simulink model "SrmMatlabZzh1"  (Simulink 7.3)
settings: Solver=ode45  StartTime=0.0  StopTime=10.0  RelTol=1e-3
libraries: powerlib x27, powerlib_extras x1
settings Model: Creator=Administrator  LastModifiedBy=Think79

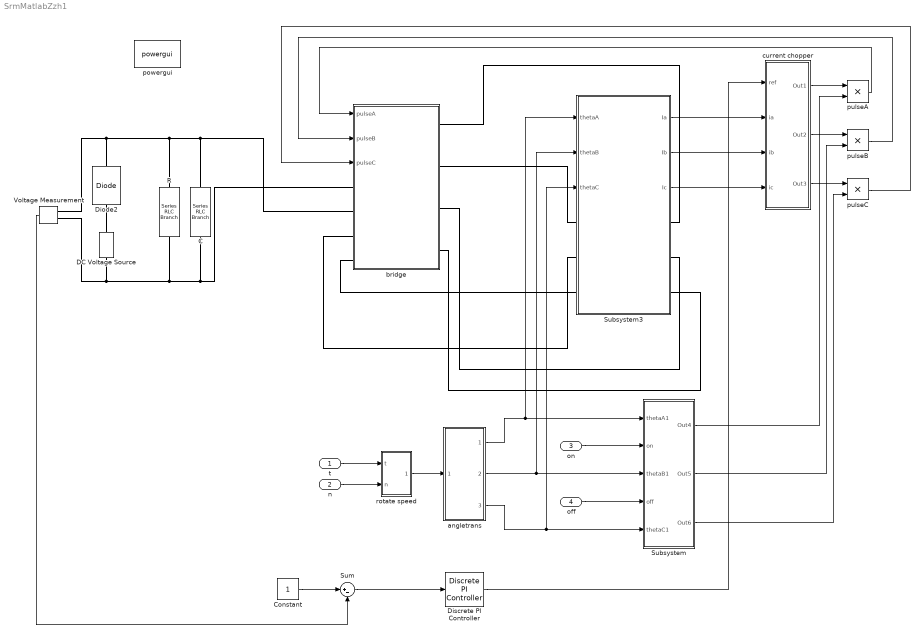
== system SrmMatlabZzh1 ==
  t : Inport  OutDataType=fixdt(1, 16)  OutScaling=2^0
  n : Inport  Port=2  OutDataType=fixdt(1, 16)  OutScaling=2^0
  on : Inport  Port=3  OutDataType=fixdt(1, 16)  OutScaling=2^0
  off : Inport  Port=4  OutDataType=fixdt(1, 16)  OutScaling=2^0
  "C " : powerlib/Elements/Series RLC Branch  DialogController=POWERSYS.PowerSysDialog  PhysicalDomain=powersysdomain  SubClassName=unknown  LeftPortType=p1  RightPortType=p1  LConnTagsString=__new0  RConnTagsString=__new0  BranchType=C  Resistance=1  Inductance=1.0  SetiL0=off  InitialCurrent=0  Capacitance=1e-3  Setx0=off  InitialVoltage=0  Measurements=None
  Constant : Constant  OutDataType=fixdt(1, 16)  OutScaling=2^0
  DC Voltage Source : powerlib/Electrical Sources/DC Voltage Source  DialogController=POWERSYS.PowerSysDialog  SystemSampleTime=-1  Amplitude=60  Measurements=None
  Diode2 : powerlib/Power Electronics/Diode  DialogController=POWERSYS.PowerSysDialog  SystemSampleTime=-1  Ron=0.001  Lon=0  Vf=0.8  IC=0  UseSnubber=off  Rs=500  Cs=250e-9  Measurements=off
  Discrete PI Controller : powerlib_extras/Discrete  Control Blocks/Discrete PI Controller  DialogController=POWERSYS.PowerSysDialog  SystemSampleTime=-1  Kp=0.1  Ki=1  Par_Limits=[1e6 -1e6]  Init=0  Ts=50e-6
  R : powerlib/Elements/Series RLC Branch  DialogController=POWERSYS.PowerSysDialog  PhysicalDomain=powersysdomain  SubClassName=unknown  LeftPortType=p1  RightPortType=p1  LConnTagsString=__new0  RConnTagsString=__new0  BranchType=R  Resistance=1  Inductance=1.0  SetiL0=off  InitialCurrent=0  Capacitance=1.0  Setx0=off  InitialVoltage=0  Measurements=None
  Subsystem : Subsystem
  Subsystem3 : Subsystem
  Sum : Sum  Inputs=|+-  OutDataType=fixdt(1, 16)  OutScaling=2^0
  Voltage Measurement : powerlib/Measurements/Voltage Measurement  DialogController=POWERSYS.PowerSysDialog  SystemSampleTime=-1  PhasorSimulation=off  OutputType=Complex  PSBequivalent=0
  angletrans : Subsystem
  bridge : Subsystem
  current chopper : Subsystem
  powergui : powerlib/powergui  Priority=1  SystemSampleTime=-1  SimulationMode=Continuous  SampleTime=50e-6  frequency=60  SPID=off  DisableSnubberDevices=off  DisableRonSwitches=off  DisableVfSwitches=off  SwTol=0  Interpol=off  frequencyindice=0  echomessages=off  HookPort=off  DisplayEquations=off  FunctionMessages=off  EnableUseOfTLC=off  x0status=blocks  RestoreLinks=warning  Frange=[0:2:500]  Ylog=off  Xlog=on  ShowGrid=off  save=off  variable=ZData  ZoomFFT=on  StartTime=0.0  cycles=1  DisplayStyle=1  fundamental=60  FreqAxis=off  MaxFrequency=1000  frequencyindicesteady=1  RmsSteady=1  display=off  Ts=0  methode=off
  pulseA : Product  OutDataType=fixdt(1, 16)  OutScaling=2^0  RndMeth=Zero
  pulseB : Product  OutDataType=fixdt(1, 16)  OutScaling=2^0  RndMeth=Zero
  pulseC : Product  OutDataType=fixdt(1, 16)  OutScaling=2^0  RndMeth=Zero
  rotate speed : Subsystem
  wires:
  Subsystem3/1(Ia) -> current chopper/2(ia)
  Subsystem3/2(Ib) -> current chopper/3(ib)
  Subsystem3/3(Ic) -> current chopper/4(ic)
  rotate speed/1(theta) -> angletrans/1(theta)
  t/1 -> rotate speed/1(t)
  n/1 -> rotate speed/2(n)
  on/1 -> Subsystem/2(on)
  off/1 -> Subsystem/4(off)
  angletrans/1(thetaA) -> Subsystem/1(thetaA1), Subsystem3/1(thetaA)
  angletrans/2(thetaB) -> Subsystem/3(thetaB1), Subsystem3/2(thetaB)
  angletrans/3(thetaC) -> Subsystem/5(thetaC1), Subsystem3/3(thetaC)
  Voltage Measurement/1 -> Sum/2
  Sum/1 -> Discrete PI Controller/1
  Constant/1 -> Sum/1
  Discrete PI Controller/1 -> current chopper/1(ref)
  Subsystem/1(Out4) -> pulseA/2
  Subsystem/3(Out6) -> pulseC/2
  Subsystem/2(Out5) -> pulseB/2
  current chopper/1(Out1) -> pulseA/1
  current chopper/2(Out2) -> pulseB/1
  current chopper/3(Out3) -> pulseC/1
  pulseB/1 -> bridge/2(pulseB)
  pulseC/1 -> bridge/3(pulseC)
  pulseA/1 -> bridge/1(pulseA)
  connections:
  Diode2/LConn1 -- DC Voltage Source/RConn1
  Diode2/RConn1 -- R/LConn1 -- "C "/RConn1 -- bridge/LConn2 -- Voltage Measurement/LConn1
  "C "/LConn1 -- bridge/LConn1 -- R/RConn1 -- DC Voltage Source/LConn1 -- Voltage Measurement/LConn2
  bridge/RConn2 -- Subsystem3/LConn1
  bridge/RConn1 -- Subsystem3/RConn1
  bridge/LConn3 -- Subsystem3/LConn2
  bridge/LConn4 -- Subsystem3/LConn3
  bridge/RConn4 -- Subsystem3/RConn3
  bridge/RConn3 -- Subsystem3/RConn2

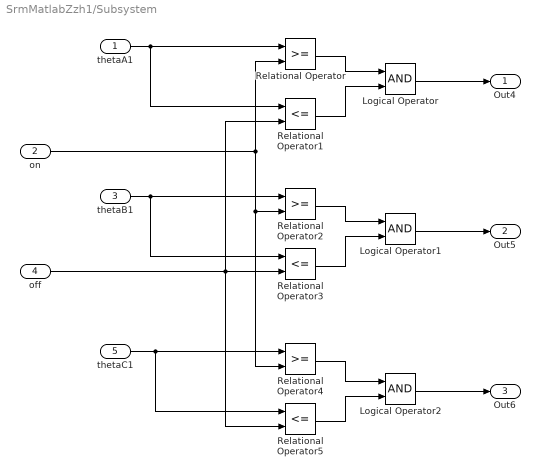
== system SrmMatlabZzh1/Subsystem ==
  thetaA1 : Inport  OutDataType=fixdt(1, 16)  OutScaling=2^0
  on : Inport  Port=2  OutDataType=fixdt(1, 16)  OutScaling=2^0
  thetaB1 : Inport  Port=3  OutDataType=fixdt(1, 16)  OutScaling=2^0
  off : Inport  Port=4  OutDataType=fixdt(1, 16)  OutScaling=2^0
  thetaC1 : Inport  Port=5  OutDataType=fixdt(1, 16)  OutScaling=2^0
  Logical Operator : Logic  AllPortsSameDT=off  OutDataTypeMode=boolean  LogicDataType=fixdt(0, 8)  OutDataTypeStr=boolean
  Logical Operator1 : Logic  AllPortsSameDT=off  OutDataTypeMode=boolean  LogicDataType=fixdt(0, 8)  OutDataTypeStr=boolean
  Logical Operator2 : Logic  AllPortsSameDT=off  OutDataTypeMode=boolean  LogicDataType=fixdt(0, 8)  OutDataTypeStr=boolean
  Relational Operator : RelationalOperator  LogicOutDataTypeMode=boolean  LogicDataType=fixdt(0, 8)  OutDataTypeStr=boolean
  Relational Operator1 : RelationalOperator  Operator=<=  LogicOutDataTypeMode=boolean  LogicDataType=fixdt(0, 8)  OutDataTypeStr=boolean
  Relational Operator2 : RelationalOperator  LogicOutDataTypeMode=boolean  LogicDataType=fixdt(0, 8)  OutDataTypeStr=boolean
  Relational Operator3 : RelationalOperator  Operator=<=  LogicOutDataTypeMode=boolean  LogicDataType=fixdt(0, 8)  OutDataTypeStr=boolean
  Relational Operator4 : RelationalOperator  LogicOutDataTypeMode=boolean  LogicDataType=fixdt(0, 8)  OutDataTypeStr=boolean
  Relational Operator5 : RelationalOperator  Operator=<=  LogicOutDataTypeMode=boolean  LogicDataType=fixdt(0, 8)  OutDataTypeStr=boolean
  Out4 : Outport  OutDataType=fixdt(1, 16)  OutScaling=2^0
  Out5 : Outport  Port=2  OutDataType=fixdt(1, 16)  OutScaling=2^0
  Out6 : Outport  Port=3  OutDataType=fixdt(1, 16)  OutScaling=2^0
  wires:
  thetaA1/1 -> Relational Operator/1, Relational Operator1/1
  thetaB1/1 -> Relational Operator2/1, Relational Operator3/1
  thetaC1/1 -> Relational Operator4/1, Relational Operator5/1
  on/1 -> Relational Operator/2, Relational Operator2/2, Relational Operator4/2
  off/1 -> Relational Operator1/2, Relational Operator3/2, Relational Operator5/2
  Relational Operator/1 -> Logical Operator/1
  Relational Operator1/1 -> Logical Operator/2
  Relational Operator2/1 -> Logical Operator1/1
  Relational Operator3/1 -> Logical Operator1/2
  Relational Operator4/1 -> Logical Operator2/1
  Relational Operator5/1 -> Logical Operator2/2
  Logical Operator/1 -> Out4/1
  Logical Operator1/1 -> Out5/1
  Logical Operator2/1 -> Out6/1

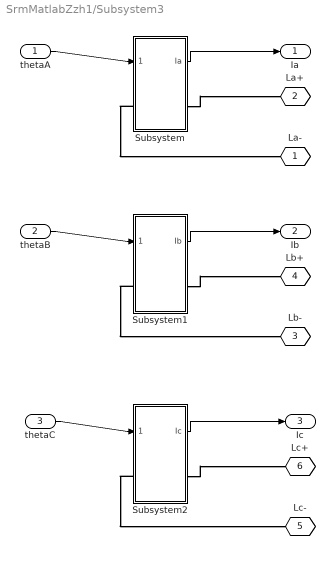
== system SrmMatlabZzh1/Subsystem3 ==
  thetaA : Inport  OutDataType=fixdt(1, 16)  OutScaling=2^0
  thetaB : Inport  Port=2  OutDataType=fixdt(1, 16)  OutScaling=2^0
  thetaC : Inport  Port=3  OutDataType=fixdt(1, 16)  OutScaling=2^0
  Subsystem : Subsystem
  Subsystem1 : Subsystem
  Subsystem2 : Subsystem
  La- : PMIOPort  Tag=PMCPort  Port=1  Side=Left
  La+ : PMIOPort  Tag=PMCPort  Port=2  Side=Right
  Lb- : PMIOPort  Tag=PMCPort  Port=3  Side=Left
  Lb+ : PMIOPort  Tag=PMCPort  Port=4  Side=Right
  Lc- : PMIOPort  Tag=PMCPort  Port=5  Side=Left
  Lc+ : PMIOPort  Tag=PMCPort  Port=6  Side=Right
  Ia : Outport  OutDataType=fixdt(1, 16)  OutScaling=2^0
  Ib : Outport  Port=2  OutDataType=fixdt(1, 16)  OutScaling=2^0
  Ic : Outport  Port=3  OutDataType=fixdt(1, 16)  OutScaling=2^0
  wires:
  thetaA/1 -> Subsystem/1(thetaA)
  Subsystem/1(Ia) -> Ia/1
  thetaB/1 -> Subsystem1/1(thetaB)
  Subsystem1/1(Ib) -> Ib/1
  thetaC/1 -> Subsystem2/1(thetaC)
  Subsystem2/1(Ic) -> Ic/1
  connections:
  Subsystem/LConn1 -- La-/RConn1
  Subsystem/RConn1 -- La+/RConn1
  Subsystem1/LConn1 -- Lb-/RConn1
  Subsystem1/RConn1 -- Lb+/RConn1
  Subsystem2/LConn1 -- Lc-/RConn1
  Subsystem2/RConn1 -- Lc+/RConn1

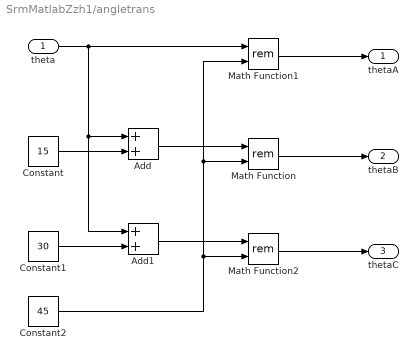
== system SrmMatlabZzh1/angletrans ==
  theta : Inport  OutDataType=fixdt(1, 16)  OutScaling=2^0
  Add : Sum  OutDataType=fixdt(1, 16)  OutScaling=2^-10
  Add1 : Sum  OutDataType=fixdt(1, 16)  OutScaling=2^-10
  Constant : Constant  Value=15  OutDataType=fixdt(1, 16)  OutScaling=2^0
  Constant1 : Constant  Value=30  OutDataType=fixdt(1, 16)  OutScaling=2^0
  Constant2 : Constant  Value=45  OutDataType=fixdt(1, 16)  OutScaling=2^0
  Math Function : Math  Operator=rem  OutDataType=fixdt(1, 16)  OutScaling=2^0  SaturateOnIntegerOverflow=on
  Math Function1 : Math  Operator=rem  OutDataType=fixdt(1, 16)  OutScaling=2^0  SaturateOnIntegerOverflow=on
  Math Function2 : Math  Operator=rem  OutDataType=fixdt(1, 16)  OutScaling=2^0  SaturateOnIntegerOverflow=on
  thetaA : Outport  OutDataType=fixdt(1, 16)  OutScaling=2^0
  thetaB : Outport  Port=2  OutDataType=fixdt(1, 16)  OutScaling=2^0
  thetaC : Outport  Port=3  OutDataType=fixdt(1, 16)  OutScaling=2^0
  wires:
  Add1/1 -> Math Function2/1
  Add/1 -> Math Function/1
  theta/1 -> Math Function1/1, Add1/1, Add/1
  Constant/1 -> Add/2
  Constant1/1 -> Add1/2
  Constant2/1 -> Math Function2/2, Math Function/2, Math Function1/2
  Math Function2/1 -> thetaC/1
  Math Function/1 -> thetaB/1
  Math Function1/1 -> thetaA/1

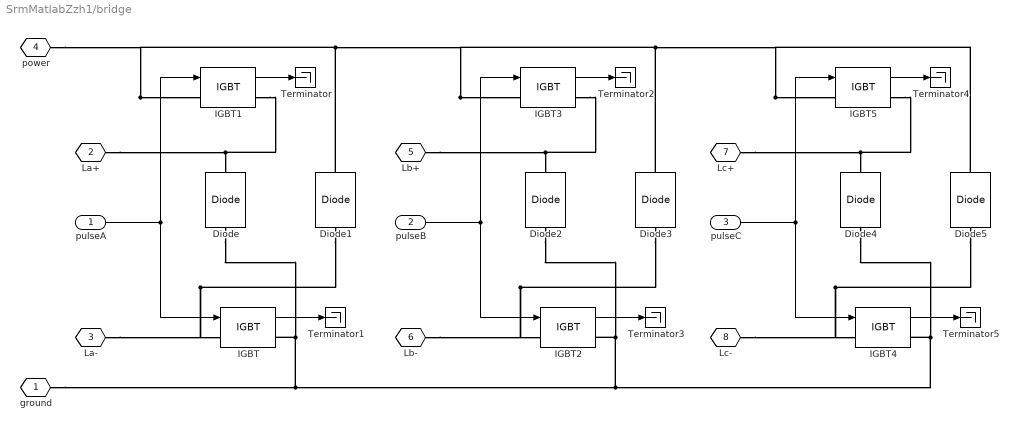
== system SrmMatlabZzh1/bridge ==
  pulseA : Inport  OutDataType=fixdt(1, 16)  OutScaling=2^0
  pulseB : Inport  Port=2  OutDataType=fixdt(1, 16)  OutScaling=2^0
  pulseC : Inport  Port=3  OutDataType=fixdt(1, 16)  OutScaling=2^0
  Diode{,1..5} (6 alike) : powerlib/Power Electronics/Diode  DialogController=POWERSYS.PowerSysDialog  SystemSampleTime=-1  Ron=0.001  Lon=0  Vf=0.8  IC=0  UseSnubber=off  Rs=500  Cs=250e-9  Measurements=off
  IGBT{,1..5} (6 alike) : powerlib/Power Electronics/IGBT  DialogController=POWERSYS.PowerSysDialog  SystemSampleTime=-1  Ron=0.001  Lon=0  Vf=1  Tf=1e-6  Tt=2e-6  IC=0  Rs=1e5  Cs=inf  Measurements=on
  Terminator{,1..5} (6 alike) : Terminator
  ground : PMIOPort  Tag=PMCPort  Port=1  Side=Left
  La+ : PMIOPort  Tag=PMCPort  Port=2  Side=Right
  La- : PMIOPort  Tag=PMCPort  Port=3  Side=Right
  power : PMIOPort  Tag=PMCPort  Port=4  Side=Left
  Lb+ : PMIOPort  Tag=PMCPort  Port=5  Side=Right
  Lb- : PMIOPort  Tag=PMCPort  Port=6  Side=Left
  Lc+ : PMIOPort  Tag=PMCPort  Port=7  Side=Right
  Lc- : PMIOPort  Tag=PMCPort  Port=8  Side=Left
  wires:
  IGBT4/1 -> Terminator5/1
  IGBT5/1 -> Terminator4/1
  pulseC/1 -> IGBT4/1, IGBT5/1
  IGBT2/1 -> Terminator3/1
  IGBT3/1 -> Terminator2/1
  pulseB/1 -> IGBT2/1, IGBT3/1
  IGBT/1 -> Terminator1/1
  IGBT1/1 -> Terminator/1
  pulseA/1 -> IGBT/1, IGBT1/1
  connections:
  Lc-/RConn1 -- IGBT4/LConn1 -- Diode5/LConn1
  Lc+/RConn1 -- IGBT5/RConn1 -- Diode4/RConn1
  Lb-/RConn1 -- IGBT2/LConn1 -- Diode3/LConn1
  Lb+/RConn1 -- IGBT3/RConn1 -- Diode2/RConn1
  Diode5/RConn1 -- IGBT5/LConn1 -- Diode3/RConn1 -- IGBT3/LConn1 -- Diode1/RConn1 -- IGBT1/LConn1 -- power/RConn1
  La-/RConn1 -- IGBT/LConn1 -- Diode1/LConn1
  La+/RConn1 -- IGBT1/RConn1 -- Diode/RConn1
  IGBT2/RConn1 -- Diode2/LConn1 -- IGBT/RConn1 -- Diode/LConn1 -- ground/RConn1 -- IGBT4/RConn1 -- Diode4/LConn1

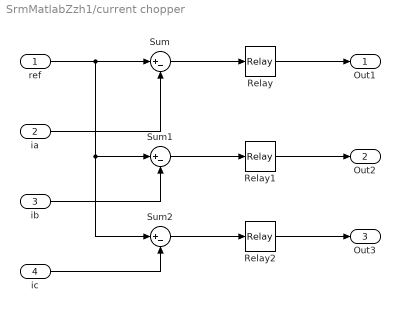
== system SrmMatlabZzh1/current chopper ==
  ref : Inport  OutDataType=fixdt(1, 16)  OutScaling=2^0
  ia : Inport  Port=2  OutDataType=fixdt(1, 16)  OutScaling=2^0
  ib : Inport  Port=3  OutDataType=fixdt(1, 16)  OutScaling=2^0
  ic : Inport  Port=4  OutDataType=fixdt(1, 16)  OutScaling=2^0
  Relay : Relay  OutDataType=fixdt(1, 16)  OutScaling=2^0
  Relay1 : Relay  OutDataType=fixdt(1, 16)  OutScaling=2^0
  Relay2 : Relay  OutDataType=fixdt(1, 16)  OutScaling=2^0
  Sum : Sum  Inputs=|+-  OutDataType=fixdt(1, 16)  OutScaling=2^0
  Sum1 : Sum  Inputs=|+-  OutDataType=fixdt(1, 16)  OutScaling=2^0
  Sum2 : Sum  Inputs=|+-  OutDataType=fixdt(1, 16)  OutScaling=2^0
  Out1 : Outport  OutDataType=fixdt(1, 16)  OutScaling=2^0
  Out2 : Outport  Port=2  OutDataType=fixdt(1, 16)  OutScaling=2^0
  Out3 : Outport  Port=3  OutDataType=fixdt(1, 16)  OutScaling=2^0
  wires:
  Relay/1 -> Out1/1
  Relay1/1 -> Out2/1
  Relay2/1 -> Out3/1
  Sum/1 -> Relay/1
  Sum1/1 -> Relay1/1
  Sum2/1 -> Relay2/1
  ref/1 -> Sum/1, Sum2/1, Sum1/1
  ia/1 -> Sum/2
  ib/1 -> Sum1/2
  ic/1 -> Sum2/2

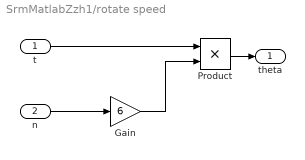
== system SrmMatlabZzh1/rotate speed ==
  t : Inport  OutDataType=fixdt(1, 16)  OutScaling=2^0
  n : Inport  Port=2  OutDataType=fixdt(1, 16)  OutScaling=2^0
  Gain : Gain  Gain=6  ParameterDataType=fixdt(1, 16)  ParameterScaling=2^0  OutDataType=fixdt(1, 16)  OutScaling=2^0
  Product : Product  OutDataType=fixdt(1, 16)  OutScaling=2^0  RndMeth=Zero
  theta : Outport
  wires:
  n/1 -> Gain/1
  Gain/1 -> Product/2
  t/1 -> Product/1
  Product/1 -> theta/1

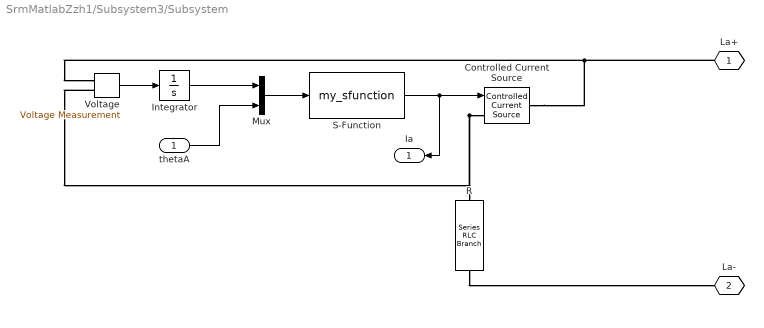
== system SrmMatlabZzh1/Subsystem3/Subsystem ==
  thetaA : Inport  OutDataType=fixdt(1, 16)  OutScaling=2^0
  Controlled Current Source : powerlib/Electrical Sources/Controlled Current Source  DialogController=POWERSYS.PowerSysDialog  SystemSampleTime=-1  Initialize=on  Source_Type=AC  Amplitude=0  Phase=0  Frequency=0  Measurements=None
  Integrator : Integrator
  Mux : Mux  Inputs=2
  R : powerlib/Elements/Series RLC Branch  DialogController=POWERSYS.PowerSysDialog  PhysicalDomain=powersysdomain  SubClassName=unknown  LeftPortType=p1  RightPortType=p1  LConnTagsString=__new0  RConnTagsString=__new0  BranchType=R  Resistance=0.0261014  Inductance=1.0  SetiL0=off  InitialCurrent=0  Capacitance=1.0  Setx0=off  InitialVoltage=0  Measurements=None
  S-Function : S-Function  FunctionName=my_sfunction  EnableBusSupport=off
  Voltage : powerlib/Measurements/Voltage Measurement  DialogController=POWERSYS.PowerSysDialog  SystemSampleTime=-1  PhasorSimulation=off  OutputType=Complex  PSBequivalent=0
  La+ : PMIOPort  Tag=PMCPort  Port=1  Side=Right
  La- : PMIOPort  Tag=PMCPort  Port=2  Side=Left
  Ia : Outport  OutDataType=fixdt(1, 16)  OutScaling=2^0
  wires:
  Mux/1 -> S-Function/1
  Integrator/1 -> Mux/1
  thetaA/1 -> Mux/2
  S-Function/1 -> Ia/1, Controlled Current Source/1
  Voltage/1 -> Integrator/1
  connections:
  Controlled Current Source/LConn1 -- Voltage/LConn2 -- R/LConn1
  La+/RConn1 -- Controlled Current Source/RConn1 -- Voltage/LConn1
  R/RConn1 -- La-/RConn1

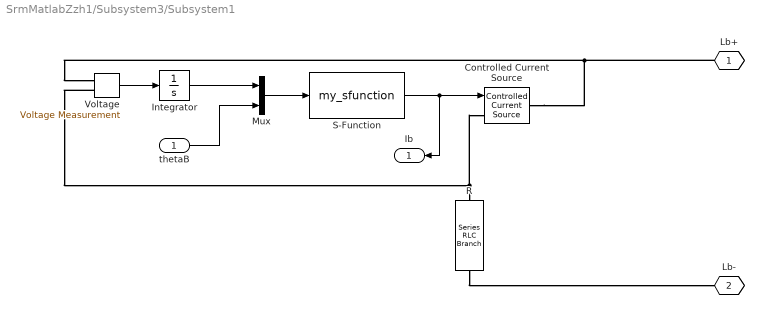
== system SrmMatlabZzh1/Subsystem3/Subsystem1 ==
  thetaB : Inport  OutDataType=fixdt(1, 16)  OutScaling=2^0
  Controlled Current Source : powerlib/Electrical Sources/Controlled Current Source  DialogController=POWERSYS.PowerSysDialog  SystemSampleTime=-1  Initialize=on  Source_Type=AC  Amplitude=0  Phase=0  Frequency=0  Measurements=None
  Integrator : Integrator
  Mux : Mux  Inputs=2
  R : powerlib/Elements/Series RLC Branch  DialogController=POWERSYS.PowerSysDialog  PhysicalDomain=powersysdomain  SubClassName=unknown  LeftPortType=p1  RightPortType=p1  LConnTagsString=__new0  RConnTagsString=__new0  BranchType=R  Resistance=0.0261014  Inductance=1.0  SetiL0=off  InitialCurrent=0  Capacitance=1.0  Setx0=off  InitialVoltage=0  Measurements=None
  S-Function : S-Function  FunctionName=my_sfunction  EnableBusSupport=off
  Voltage : powerlib/Measurements/Voltage Measurement  DialogController=POWERSYS.PowerSysDialog  SystemSampleTime=-1  PhasorSimulation=off  OutputType=Complex  PSBequivalent=0
  Lb+ : PMIOPort  Tag=PMCPort  Port=1  Side=Right
  Lb- : PMIOPort  Tag=PMCPort  Port=2  Side=Left
  Ib : Outport  OutDataType=fixdt(1, 16)  OutScaling=2^0
  wires:
  Mux/1 -> S-Function/1
  Integrator/1 -> Mux/1
  thetaB/1 -> Mux/2
  S-Function/1 -> Ib/1, Controlled Current Source/1
  Voltage/1 -> Integrator/1
  connections:
  Voltage/LConn2 -- Controlled Current Source/LConn1 -- R/LConn1
  Controlled Current Source/RConn1 -- Lb+/RConn1 -- Voltage/LConn1
  R/RConn1 -- Lb-/RConn1

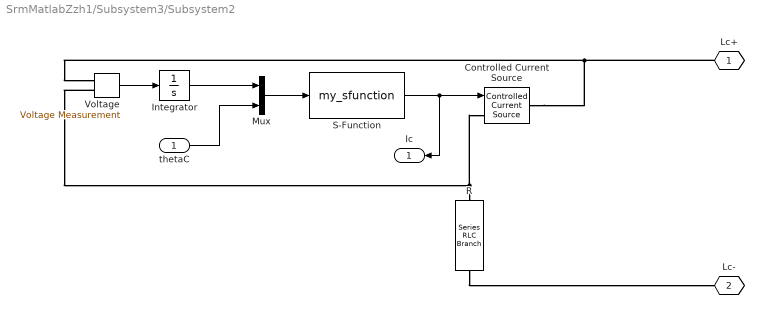
== system SrmMatlabZzh1/Subsystem3/Subsystem2 ==
  thetaC : Inport  OutDataType=fixdt(1, 16)  OutScaling=2^0
  Controlled Current Source : powerlib/Electrical Sources/Controlled Current Source  DialogController=POWERSYS.PowerSysDialog  SystemSampleTime=-1  Initialize=on  Source_Type=AC  Amplitude=0  Phase=0  Frequency=0  Measurements=None
  Integrator : Integrator
  Mux : Mux  Inputs=2
  R : powerlib/Elements/Series RLC Branch  DialogController=POWERSYS.PowerSysDialog  PhysicalDomain=powersysdomain  SubClassName=unknown  LeftPortType=p1  RightPortType=p1  LConnTagsString=__new0  RConnTagsString=__new0  BranchType=R  Resistance=0.0261014  Inductance=1.0  SetiL0=off  InitialCurrent=0  Capacitance=1.0  Setx0=off  InitialVoltage=0  Measurements=None
  S-Function : S-Function  FunctionName=my_sfunction  EnableBusSupport=off
  Voltage : powerlib/Measurements/Voltage Measurement  DialogController=POWERSYS.PowerSysDialog  SystemSampleTime=-1  PhasorSimulation=off  OutputType=Complex  PSBequivalent=0
  Lc+ : PMIOPort  Tag=PMCPort  Port=1  Side=Right
  Lc- : PMIOPort  Tag=PMCPort  Port=2  Side=Left
  Ic : Outport  OutDataType=fixdt(1, 16)  OutScaling=2^0
  wires:
  Mux/1 -> S-Function/1
  Integrator/1 -> Mux/1
  thetaC/1 -> Mux/2
  S-Function/1 -> Ic/1, Controlled Current Source/1
  Voltage/1 -> Integrator/1
  connections:
  Voltage/LConn2 -- Controlled Current Source/LConn1 -- R/LConn1
  Controlled Current Source/RConn1 -- Lc+/RConn1 -- Voltage/LConn1
  R/RConn1 -- Lc-/RConn1
